simulink model "Assignment_2_PacemakerProj"  (R2022b)
settings: Solver=FixedStepAuto  StartTime=0.0  StopTime=100  FixedStep=1e-3  RelTol=1e-3  EnableMultiTasking=on
undefined symbols (not defined in the file): D0, D1, D10, D11, D12, D13, D2, D3, D4, D5, D6, D7, D8, D9, PTA0, PTA1, PTA2, PTB23, PTB9, PTC16, PTC17, PTC2, PTC3, PTC4, PTD0, PTD1, PTD2, PTD3
libraries: frdmk64flib x24, etargetslib x3, simulink x3
settings Model: ExtModeTrigDuration=5  Creator=varun  LastModifiedBy=lupas
settings OptimizationCC: EnhancedBackFolding=on  PassReuseOutputArgsAs=Individual arguments  ZeroExternalMemoryAtStartup=off  ZeroInternalMemoryAtStartup=off  MaxStackSize=64  OptimizeBlockOrder=speed  DifferentSizesBufferReuse=on  OptimizationCustomize=off  EfficientTunableParamExpr=on
settings DebuggingCC: ParameterTunabilityLossMsg=error
settings HardwareCC: ProdBitPerPointer=32  ProdBitPerSizeT=32  ProdBitPerPtrDiffT=32  ProdLargestAtomicInteger=Long  ProdLargestAtomicFloat=Double  ProdWordSize=32  ProdHWDeviceType=ARM Compatible->ARM Cortex
settings SFSimCC: MATLABDynamicMemAlloc=off
settings RTWCC: Description=Embedded Coder  SystemTargetFile=ert.tlc  HardwareBoard=NXP FRDM-K64F  TLCOptions="-aInlineSetEventsForThisBaseRateFcn=TLC_FALSE -aSuppressMultiTaskScheduler=TLC_FALSE  -aRateBasedStepFcn=0"  TemplateMakefile=ert_default_tmf  Toolchain=GNU Tools for ARM Embedded Processors
settings CodeAppCC: ForceParamTrailComments=on  IgnoreCustomStorageClasses=off  OperatorAnnotations=on  SimulinkDataObjDesc=on  SFDataObjDesc=on  InsertBlockDesc=on
settings ERTTargetCC: ExtModeTransport=4  ExtModeMexFile=sendToCommService

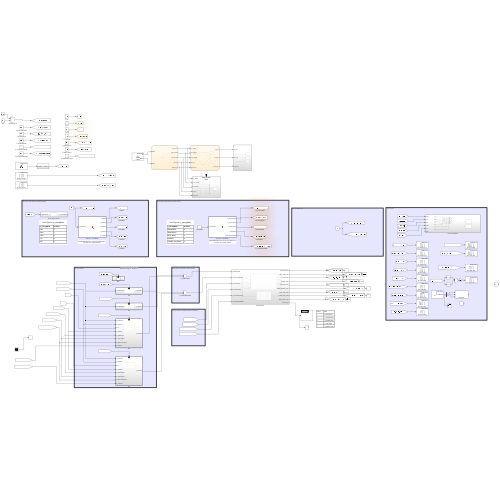
[thumbnail: Simulink's stored preview of the top-level diagram]
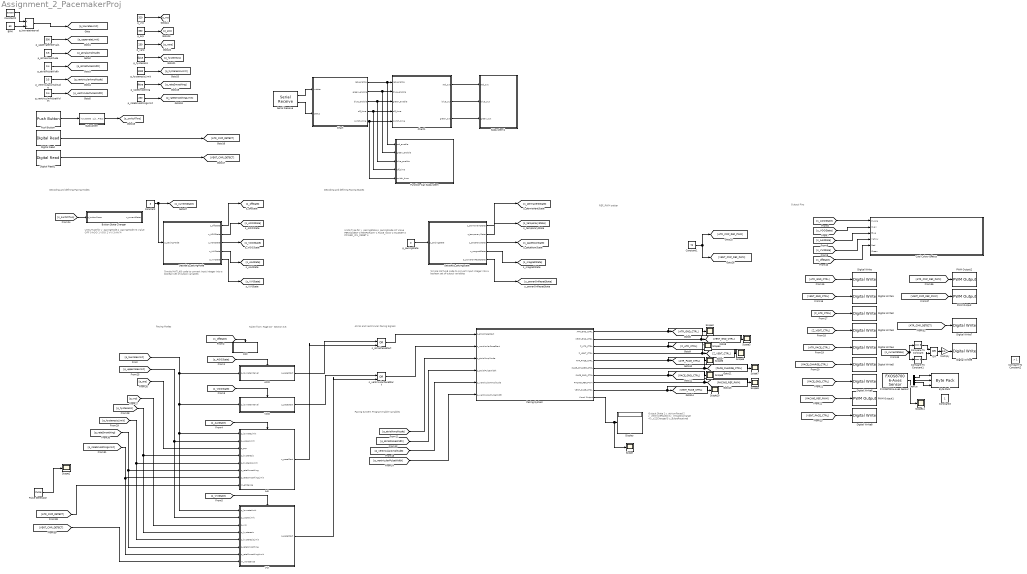
== system Assignment_2_PacemakerProj ==
  note: REF_PWM setter
  note: Output Pins
  note: Pacing System Programmable Variables
  note: Output
      | State
      |
      | 1
      | y_atriumPaced
      |
      | 2
      | y_ventriclePaced
      |
      | 3
      | y_initialDischarge
      |
      | 4
      | y_c22Charged
      |
      | 5
      | y_pulseReceived
  note: Atrial and Ventricular Pacing Signals
  note: Decoding and defining Pacing States
  note: Decoding and defining Pacing Modes
  note: Simple MATLAB code to convert input integer into a boolean set of output variables
  note: Taken from: Page 16 - Section 3.5
  note: Units/Type for y_pacingMode
      |
      | p_pacingMode
      | Int Value
      |
      | OFF
      | 0
      |
      | AOO
      | 1
      |
      | VOO
      | 2
      |
      | VVI
      | 3
      |
      | AAI
      | 4
  note: Pacing Modes
  note: Units/Type for y_pacingState
      |
      | p_pacingMode
      | Int Value
      |
      | PERMANENT
      | 0
      |
      | TEMPORARY
      | 1
      |
      | PACE_NOW
      | 2
      |
      | MAGNET
      | 3
      |
      | POWER_ON_RESET
      | 4
  note: Simple MATLAB code to convert input integer into a boolean set of output variables
  AAI : Subsystem
  AOO : Subsystem
  BPM : Constant  Value=60
  Button State Changer : Subsystem
  Byte Pack : etargetslib/Byte Pack  datatypes={'double', 'double', 'double'}  byteAlign=1
  Chart : Stateflow chart  TreatAsAtomicUnit=on
  Chart1 : Stateflow chart  TreatAsAtomicUnit=on
  Compare To Constant : simulink/Logic and Bit Operations/Compare To Constant  relop===  const=3  OutDataTypeStr=boolean
  Compare To Constant1 : simulink/Logic and Bit Operations/Compare To Constant  relop===  const=4  OutDataTypeStr=boolean
  Compare To Constant2 : simulink/Logic and Bit Operations/Compare To Constant  relop=>  const=1  OutDataTypeStr=boolean
  Constant : Constant  Value=3
  Constant1 : Constant  Value=70
  Constant2 : Constant  Value=60000
  Constant3 : Constant
  Cool Colour Effects : Subsystem
  Decode p_pacingMode : MATLAB Function  TreatAsAtomicUnit=on
  Decode p_pacingState : MATLAB Function  TreatAsAtomicUnit=on
  Demux : Demux  Outputs=3
  Digital Read : frdmk64flib/Digital Read  Whichpin=PTC16 (D0)  SampleTime=-1
  Digital Read1 : frdmk64flib/Digital Read  Whichpin=PTC17 (D1)  SampleTime=-1
  Digital Write : frdmk64flib/Digital Write  Whichpin=PTD2 (D11)
  Digital Write1 : frdmk64flib/Digital Write  Whichpin=PTD3 (D12)
  Digital Write2 : frdmk64flib/Digital Write  Whichpin=PTB23 (D4)
  Digital Write3 : frdmk64flib/Digital Write  Whichpin=PTC3 (D7)
  Digital Write4 : frdmk64flib/Digital Write  Whichpin=PTA0 (D8)
  Digital Write5 : frdmk64flib/Digital Write  Whichpin=PTB9 (D2)
  Digital Write6 : frdmk64flib/Digital Write  Whichpin=PTD0 (D10)
  Digital Write7 : frdmk64flib/Digital Write  Whichpin=RED_LED
  Digital Write8 : frdmk64flib/Digital Write  Whichpin=PTC4 (D9)
  Digital Write9 : frdmk64flib/Digital Write  Whichpin=PTD1 (D13)
  Display : Display
  FXOS8700 6-Axes Sensor : frdmk64flib/FXOS8700 6-Axes Sensor  Activesensor=Accelerometer only  ODR=400Hz  HybridODR=400Hz  Accelfullrange=-4g to +4g  SampleTime=-1
  Function-Call Subsystem : Subsystem  TreatAsAtomicUnit=on
  Multiply : Gain  Gain=3.3  OutDataTypeStr=double
  OFF : Subsystem
  OR : Logic  Operator=OR  IconShape=distinctive  AllPortsSameDT=off  OutDataTypeStr=boolean
  PWM Output : frdmk64flib/PWM Output  Whichpin=PTA1 (D3)  InitialFrequency=2000  InitialDutyCycle=50
  PWM Output1 : frdmk64flib/PWM Output  Whichpin=PTA2 (D5)  InitialFrequency=2000  InitialDutyCycle=50
  PWM Output2 : frdmk64flib/PWM Output  Whichpin=PTC2 (D6)  InitialFrequency=2000  InitialDutyCycle=50
  Pacing System : Subsystem
  Pulse Generator : DiscretePulseGenerator  PulseType=Time based  Amplitude=3.5  PulseWidth=0.5
  Push Button : frdmk64flib/Push Button  Whichswitch=SW2  SampleTime1=-1
  Scope{,1..11} (12 alike) : Scope
  Serial Receive : frdmk64flib/Serial Receive  SCIModule=0  Baudrate=uint32(9600)  Parity=None  StopBits=1  HardwareFlowControl=None  ByteOrder=LittleEndian  DataType=uint8  DataLength=11  BlockingMode=off  OutputStatus=on  SampleTime=0.1
  Subsystem : Subsystem
  Subsystem1 : Subsystem
  VOO : Subsystem
  VVI : Subsystem
  p_arp : Constant  Value=350  OutDataTypeStr=int16
  p_atrialAmplitude : Constant  Value=3.5  OutDataTypeStr=double
  p_atrialPulseWidth : Constant  Value=0.4  OutDataTypeStr=double
  p_hysteresis : Constant  Value=false  OutDataTypeStr=boolean
  p_hysteresisLimit : Constant  Value=1000  OutDataTypeStr=int16
  p_lowrateInterval : Product  Inputs=*/
  p_pacingState : Constant  Value=0
  p_rateSmoothing : Constant  Value=false  OutDataTypeStr=boolean
  p_rateSmoothingLimit : Constant  Value=250  OutDataTypeStr=uint16
  p_upperrateInterval1 : Constant  Value=500  OutDataTypeStr=int16
  p_varp : Constant  Value=250  OutDataTypeStr=int16
  p_ventricularAmplitude : Constant  Value=3.5  OutDataTypeStr=double
  p_ventricularPulseWidth : Constant  Value=0.4  OutDataTypeStr=double
  p_vrp : Constant  Value=320  OutDataTypeStr=int16
  s_atrialPaceStart : Logic  Operator=OR  IconShape=distinctive  AllPortsSameDT=off  OutDataTypeStr=boolean
  s_ventricularPaceStart : Logic  Operator=OR  IconShape=distinctive  AllPortsSameDT=off  OutDataTypeStr=boolean
  wires:
  [s_offState] -> OFF/Enable
  Decode p_pacingMode/1(s_offState) -> [s_offState]
  Decode p_pacingMode/2(s_AOOState) -> [s_AOOState]
  Decode p_pacingMode/4(s_AAIState) -> [s_AAIState]
  Decode p_pacingMode/5(S_VVIState) -> [s_VVIState]
  Decode p_pacingMode/3(s_VOOState) -> [s_VOOState]
  p_pacingState/1 -> Decode p_pacingState/1(p_pacingState)
  Decode p_pacingState/1(s_permanentState) -> [s_permanentState]
  Decode p_pacingState/2(s_temporaryState) -> [s_temporaryState]
  Decode p_pacingState/3(s_paceNowState) -> [s_paceNowState]
  Decode p_pacingState/4(s_magnetState) -> [s_magnetState]
  Decode p_pacingState/5(S_powerOnResetState) -> [s_powerOnResetState]
  AAI/1(s_paceStart) -> s_atrialPaceStart/2
  VVI/1(s_paceStart) -> s_ventricularPaceStart/2
  [s_AAIState] -> AAI/Enable
  [s_VVIState] -> VVI/Enable
  [s_AOOState] -> Cool Colour Effects/1(Purple)
  [s_VOOState] -> Cool Colour Effects/2(Cyan)
  [s_AAIState] -> Cool Colour Effects/3(Blue)
  [s_VVIState] -> Cool Colour Effects/4(Yellow)
  [s_offState] -> Cool Colour Effects/5(Red)
  p_upperrateInterval1/1 -> [p_upperrateLimit]
  p_atrialAmplitude/1 -> [p_atrialAmplitude]
  p_atrialPulseWidth/1 -> [p_atrialPulseWidth]
  p_ventricularAmplitude/1 -> [p_ventricularAmplitude]
  p_ventricularPulseWidth/1 -> [p_ventricularPulseWidth]
  s_atrialPaceStart/1 -> Pacing System/1(s_atrialPaceStart)
  [p_atrialAmplitude] -> Pacing System/3(p_atrialAmplitude)
  [p_atrialPulseWidth] -> Pacing System/4(p_atrialPulseWidth)
  [p_ventricularAmplitude] -> Pacing System/5(p_ventricularAmplitude)
  [p_ventricularPulseWidth] -> Pacing System/6(p_ventricularPulseWidth)
  s_ventricularPaceStart/1 -> Pacing System/2(s_ventricularPaceStart)
  Pacing System/1(ATR_GND_CTRL) -> [ATR_GND_CTRL], Scope2/1
  Pacing System/3(Z_ATR_CTRL) -> [Z_ATR_CTRL], Scope4/1
  Pacing System/2(VENT_GND_CTRL) -> [VENT_GND_CTRL], Scope3/1
  Pacing System/4(Z_VENT_CTRL) -> Scope5/1, [Z_VENT_CTRL]
  Pacing System/6(PACE_CHARGE_CTRL) -> Scope7/1, [PACE_CHARGE_CTRL]
  Pacing System/5(ATR_PACE_CTRL) -> [ATR_PACE_CTRL], Scope6/1
  Pacing System/7(PACE_GND_CTRL) -> Scope8/1, [PACE_GND_CTRL]
  Pacing System/9(VENT_PACE_CTRL) -> [VENT_PACE_CTRL], Scope10/1
  Pacing System/8(PACING_REF_PWM) -> Scope9/1, [PACING_REF_PWM]
  Pacing System/10(Visual Output) -> Scope/1, Display/1
  [VENT_PACE_CTRL] -> Digital Write8/1
  [PACING_REF_PWM] -> PWM Output1/1
  [PACE_GND_CTRL] -> Digital Write6/1
  [PACE_CHARGE_CTRL] -> Digital Write5/1
  [ATR_PACE_CTRL] -> Digital Write4/1
  [Z_VENT_CTRL] -> Digital Write3/1
  [Z_ATR_CTRL] -> Digital Write2/1
  [VENT_GND_CTRL] -> Digital Write1/1
  [ATR_GND_CTRL] -> Digital Write/1
  Push Button/1 -> Subsystem/1(inputState)
  Subsystem/1(s_buttonPress) -> [s_switchTwo]
  [s_switchTwo] -> Button State Changer/1(s_buttonPress)
  [s_AOOState] -> AOO/Enable
  [s_VOOState] -> VOO/Enable
  [p_lowrateLimit] -> VVI/1(p_lowrateLimit), AAI/1(p_lowrateLimit), VOO/1(p_lowrateInterval), AOO/1(p_lowrateInterval)
  AOO/1(s_paceStart) -> s_atrialPaceStart/1
  VOO/1(s_paceStart) -> s_ventricularPaceStart/1
  p_rateSmoothingLimit/1 -> [p_rateSmoothingLimit]
  p_rateSmoothing/1 -> [p_rateSmoothing]
  p_hysteresisLimit/1 -> [p_hysteresisLimit]
  p_hysteresis/1 -> [p_hysteresis]
  p_vrp/1 -> [p_vrp]
  p_arp/1 -> [p_arp]
  p_varp/1 -> [p_varp]
  [p_upperrateLimit] -> VVI/2(p_upperLimit), AAI/2(p_upperLimit)
  [p_arp] -> AAI/3(p_arp)
  [p_vrp] -> VVI/3(p_vrp)
  [p_hysteresis] -> VVI/4(p_hysteresis), AAI/4(p_hysteresis)
  [p_hysteresisLimit] -> VVI/5(p_hysteresisLimit), AAI/5(p_hystersisLimit)
  [p_rateSmoothing] -> VVI/6(p_rateSmoothing), AAI/6(p_rateSmoothing)
  [p_rateSmoothingLimit] -> VVI/7(p_rateSmoothingLimit), AAI/7(p_rateSmoothingLimit)
  Digital Read/1 -> [ATR_CMP_DETECT]
  Digital Read1/1 -> [VENT_CMP_DETECT]
  [ATR_CMP_REF_PWM] -> PWM Output2/1
  [VENT_CMP_REF_PWM] -> PWM Output/1
  [VENT_CMP_DETECT] -> VVI/8(m_ventSense)
  BPM/1 -> p_lowrateInterval/2
  p_lowrateInterval/1 -> [p_lowrateLimit]
  Constant2/1 -> p_lowrateInterval/1
  Constant1/1 -> [ATR_CMP_REF_PWM], [VENT_CMP_REF_PWM]
  Constant/1 -> Decode p_pacingMode/1(p_pacingMode), [s_currentState]
  OR/1 -> Multiply/1
  Compare To Constant/1 -> OR/1
  Compare To Constant1/1 -> OR/2
  Multiply/1 -> Digital Write9/1
  Pulse Generator/1 -> Scope1/1
  [s_currentState] -> Compare To Constant1/1, Compare To Constant/1
  [ATR_CMP_DETECT] -> AAI/8(m_atrSense)
  Demux/1 -> Byte Pack/1
  Demux/2 -> Byte Pack/2
  Demux/3 -> Byte Pack/3
  FXOS8700 6-Axes Sensor/1 -> Scope11/1
  [ATR_CMP_DETECT] -> Digital Write7/1
  Serial Receive/1 -> Chart/1(rxdata)
  Serial Receive/2 -> Chart/2(status)
  Chart/1(red_enable) -> Function-Call Subsystem/1(red_enable), Chart1/1(red_enable)
  Chart/2(green_enable) -> Function-Call Subsystem/2(green_enable), Chart1/2(blue_enable)
  Chart/3(blue_enable) -> Function-Call Subsystem/3(blue_enable), Chart1/3(green_enable)
  Chart/4(off_time) -> Function-Call Subsystem/4(off_time), Chart1/4(off_time)
  Chart/5(switch_time) -> Function-Call Subsystem/5(switch_time), Chart1/5(switch_time)
  Chart1/1(red_out) -> Subsystem1/1(red_out)
  Chart1/2(blue_out) -> Subsystem1/2(blue_out)
  Chart1/3(green_out) -> Subsystem1/3(green_out)

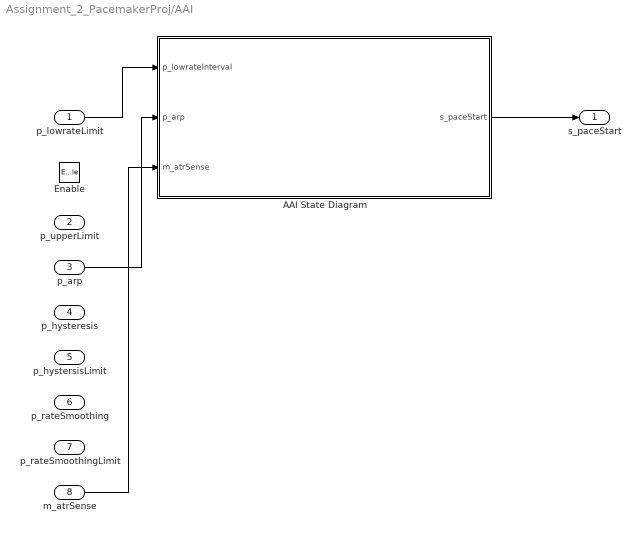
== system Assignment_2_PacemakerProj/AAI ==
  p_lowrateLimit : Inport
  p_upperLimit : Inport  Port=2
  p_arp : Inport  Port=3
  p_hysteresis : Inport  Port=4
  p_hystersisLimit : Inport  Port=5
  p_rateSmoothing : Inport  Port=6
  p_rateSmoothingLimit : Inport  Port=7
  m_atrSense : Inport  Port=8
  Enable : EnablePort
  AAI State Diagram : Stateflow chart  TreatAsAtomicUnit=on
  s_paceStart : Outport
  wires:
  p_lowrateLimit/1 -> AAI State Diagram/1(p_lowrateInterval)
  AAI State Diagram/1(s_paceStart) -> s_paceStart/1
  m_atrSense/1 -> AAI State Diagram/3(m_atrSense)
  p_arp/1 -> AAI State Diagram/2(p_arp)

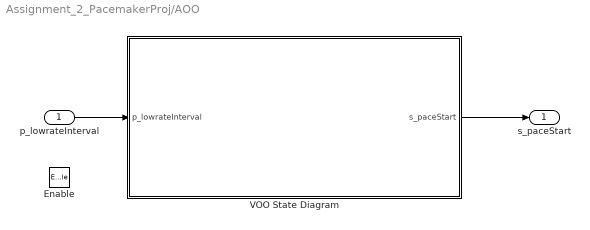
== system Assignment_2_PacemakerProj/AOO ==
  p_lowrateInterval : Inport
  Enable : EnablePort
  VOO State Diagram : Stateflow chart  TreatAsAtomicUnit=on
  s_paceStart : Outport
  wires:
  p_lowrateInterval/1 -> VOO State Diagram/1(p_lowrateInterval)
  VOO State Diagram/1(s_paceStart) -> s_paceStart/1

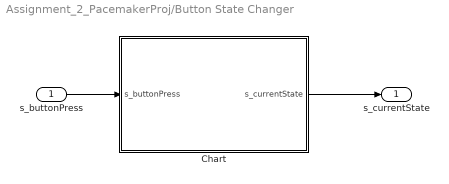
== system Assignment_2_PacemakerProj/Button State Changer ==
  s_buttonPress : Inport  OutDataTypeStr=boolean
  Chart : Stateflow chart  TreatAsAtomicUnit=on
  s_currentState : Outport
  wires:
  s_buttonPress/1 -> Chart/1(s_buttonPress)
  Chart/1(s_currentState) -> s_currentState/1

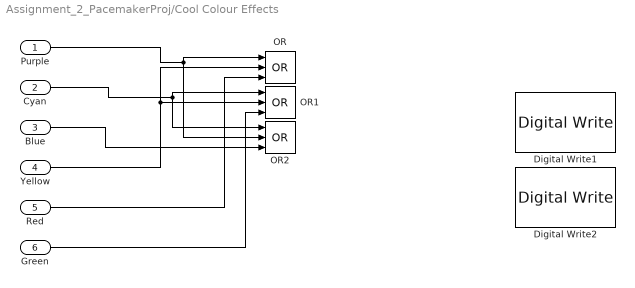
== system Assignment_2_PacemakerProj/Cool Colour Effects ==
  Purple : Inport
  Cyan : Inport  Port=2
  Blue : Inport  Port=3
  Yellow : Inport  Port=4
  Red : Inport  Port=5
  Green : Inport  Port=6
  Digital Write1 : frdmk64flib/Digital Write  Whichpin=GREEN_LED
  Digital Write2 : frdmk64flib/Digital Write  Whichpin=BLUE_LED
  OR : Logic  Operator=OR  Inputs=3  IconShape=distinctive  AllPortsSameDT=off  OutDataTypeStr=boolean
  OR1 : Logic  Operator=OR  Inputs=3  IconShape=distinctive  AllPortsSameDT=off  OutDataTypeStr=boolean
  OR2 : Logic  Operator=OR  Inputs=3  IconShape=distinctive  AllPortsSameDT=off  OutDataTypeStr=boolean
  wires:
  Blue/1 -> OR2/3
  Cyan/1 -> OR2/1, OR1/1
  Purple/1 -> OR2/2, OR/1
  Yellow/1 -> OR1/2, OR/2
  Red/1 -> OR/3
  Green/1 -> OR1/3

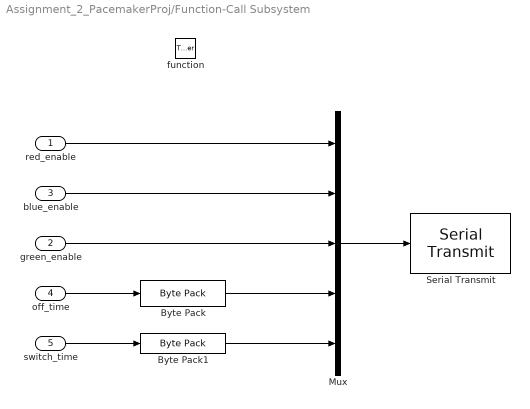
== system Assignment_2_PacemakerProj/Function-Call Subsystem ==
  red_enable : Inport
  green_enable : Inport  Port=2
  blue_enable : Inport  Port=3
  off_time : Inport  Port=4
  switch_time : Inport  Port=5
  function : TriggerPort  TriggerType=function-call  IsSimulinkFunction=on  FunctionName=send_params  VariantControl=(inherit)
  Byte Pack : etargetslib/Byte Pack  datatypes={'single'}  byteAlign=1
  Byte Pack1 : etargetslib/Byte Pack  datatypes={'uint16'}  byteAlign=1
  Mux : Mux  Inputs=5
  Serial Transmit : frdmk64flib/Serial Transmit  SCIModule=0  Baudrate=uint32(9600)  Parity=None  StopBits=1  HardwareFlowControl=None  ByteOrder=LittleEndian  BlockingMode=on  OutputStatus=off
  wires:
  switch_time/1 -> Byte Pack1/1
  green_enable/1 -> Mux/3
  blue_enable/1 -> Mux/2
  Mux/1 -> Serial Transmit/1
  off_time/1 -> Byte Pack/1
  Byte Pack1/1 -> Mux/5
  Byte Pack/1 -> Mux/4
  red_enable/1 -> Mux/1

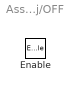
== system Assignment_2_PacemakerProj/OFF ==
  Enable : EnablePort

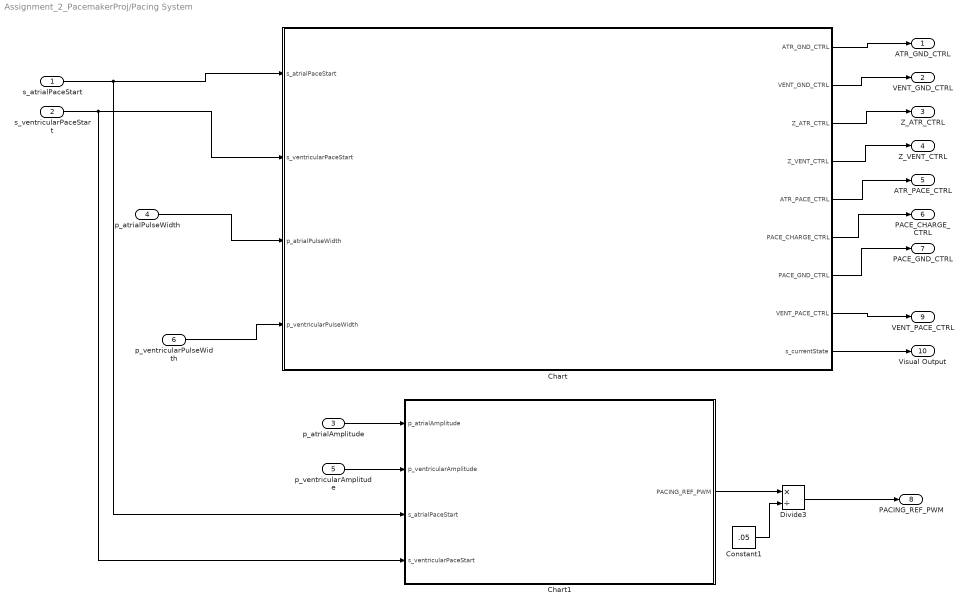
== system Assignment_2_PacemakerProj/Pacing System ==
  s_atrialPaceStart : Inport
  s_ventricularPaceStart : Inport  Port=2
  p_atrialAmplitude : Inport  Port=3
  p_atrialPulseWidth : Inport  Port=4
  p_ventricularAmplitude : Inport  Port=5  OutDataTypeStr=double
  p_ventricularPulseWidth : Inport  Port=6  OutDataTypeStr=double
  Chart : Stateflow chart  TreatAsAtomicUnit=on
  Chart1 : Stateflow chart  TreatAsAtomicUnit=on
  Constant1 : Constant  Value=.05  OutDataTypeStr=double
  Divide3 : Product  Inputs=*/
  ATR_GND_CTRL : Outport
  VENT_GND_CTRL : Outport  Port=2
  Z_ATR_CTRL : Outport  Port=3
  Z_VENT_CTRL : Outport  Port=4
  ATR_PACE_CTRL : Outport  Port=5
  PACE_CHARGE_CTRL : Outport  Port=6
  PACE_GND_CTRL : Outport  Port=7
  PACING_REF_PWM : Outport  Port=8
  VENT_PACE_CTRL : Outport  Port=9
  Visual Output : Outport  Port=10
  wires:
  s_atrialPaceStart/1 -> Chart1/3(s_atrialPaceStart), Chart/1(s_atrialPaceStart)
  s_ventricularPaceStart/1 -> Chart1/4(s_ventricularPaceStart), Chart/2(s_ventricularPaceStart)
  p_atrialPulseWidth/1 -> Chart/3(p_atrialPulseWidth)
  Chart/1(ATR_GND_CTRL) -> ATR_GND_CTRL/1
  Chart/2(VENT_GND_CTRL) -> VENT_GND_CTRL/1
  Chart/3(Z_ATR_CTRL) -> Z_ATR_CTRL/1
  Chart/4(Z_VENT_CTRL) -> Z_VENT_CTRL/1
  Chart/5(ATR_PACE_CTRL) -> ATR_PACE_CTRL/1
  Chart/6(PACE_CHARGE_CTRL) -> PACE_CHARGE_CTRL/1
  Chart/7(PACE_GND_CTRL) -> PACE_GND_CTRL/1
  Chart/8(VENT_PACE_CTRL) -> VENT_PACE_CTRL/1
  Chart/9(s_currentState) -> Visual Output/1
  p_ventricularPulseWidth/1 -> Chart/4(p_ventricularPulseWidth)
  p_ventricularAmplitude/1 -> Chart1/2(p_ventricularAmplitude)
  p_atrialAmplitude/1 -> Chart1/1(p_atrialAmplitude)
  Chart1/1(PACING_REF_PWM) -> Divide3/1
  Constant1/1 -> Divide3/2
  Divide3/1 -> PACING_REF_PWM/1

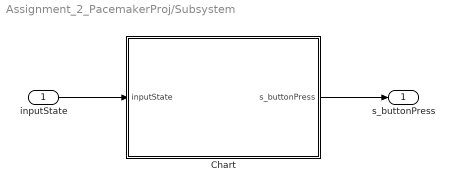
== system Assignment_2_PacemakerProj/Subsystem ==
  inputState : Inport
  Chart : Stateflow chart  TreatAsAtomicUnit=on
  s_buttonPress : Outport
  wires:
  inputState/1 -> Chart/1(inputState)
  Chart/1(s_buttonPress) -> s_buttonPress/1

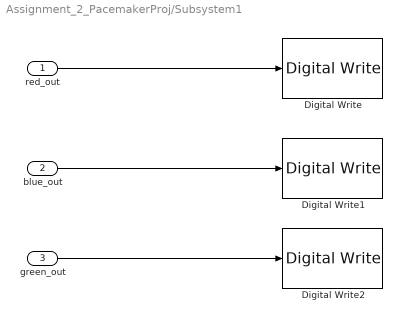
== system Assignment_2_PacemakerProj/Subsystem1 ==
  red_out : Inport
  blue_out : Inport  Port=2
  green_out : Inport  Port=3
  Digital Write : frdmk64flib/Digital Write  Whichpin=RED_LED
  Digital Write1 : frdmk64flib/Digital Write  Whichpin=GREEN_LED
  Digital Write2 : frdmk64flib/Digital Write  Whichpin=BLUE_LED
  wires:
  red_out/1 -> Digital Write/1
  blue_out/1 -> Digital Write1/1
  green_out/1 -> Digital Write2/1

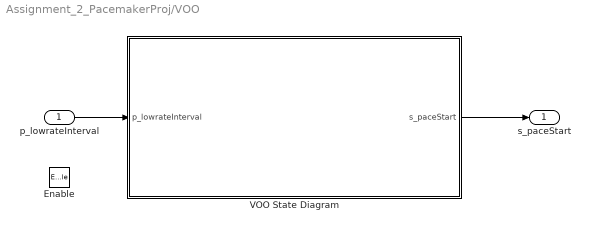
== system Assignment_2_PacemakerProj/VOO ==
  p_lowrateInterval : Inport
  Enable : EnablePort
  VOO State Diagram : Stateflow chart  TreatAsAtomicUnit=on
  s_paceStart : Outport
  wires:
  p_lowrateInterval/1 -> VOO State Diagram/1(p_lowrateInterval)
  VOO State Diagram/1(s_paceStart) -> s_paceStart/1

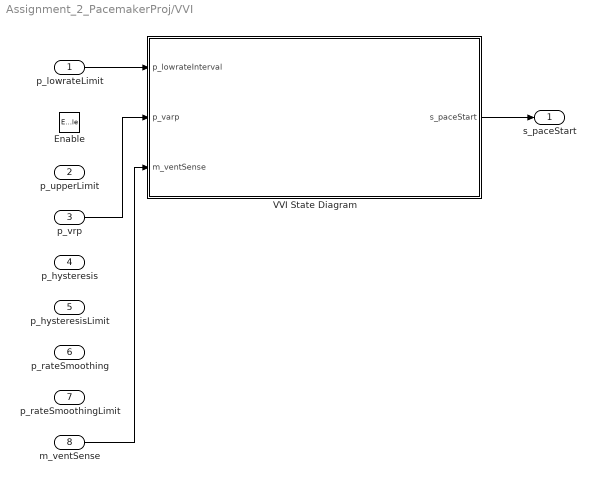
== system Assignment_2_PacemakerProj/VVI ==
  p_lowrateLimit : Inport
  p_upperLimit : Inport  Port=2
  p_vrp : Inport  Port=3
  p_hysteresis : Inport  Port=4
  p_hysteresisLimit : Inport  Port=5
  p_rateSmoothing : Inport  Port=6
  p_rateSmoothingLimit : Inport  Port=7
  m_ventSense : Inport  Port=8
  Enable : EnablePort
  VVI State Diagram : Stateflow chart  TreatAsAtomicUnit=on
  s_paceStart : Outport
  wires:
  p_lowrateLimit/1 -> VVI State Diagram/1(p_lowrateInterval)
  VVI State Diagram/1(s_paceStart) -> s_paceStart/1
  p_vrp/1 -> VVI State Diagram/2(p_varp)
  m_ventSense/1 -> VVI State Diagram/3(m_ventSense)

== matlab function Assignment_2_PacemakerProj/Decode p_pacingState ==
  data: p_pacingState input; s_permanentState output; s_temporaryState output; s_paceNowState output; s_magnetState output; S_powerOnResetState output
function [s_permanentState,s_temporaryState, s_paceNowState, s_magnetState, S_powerOnResetState] = decodeInputInteger(p_pacingState)

stateList = zeros(1,5);

stateList(p_pacingState + 1) = 1;

s_permanentState = stateList(1);
s_temporaryState = stateList(2);
s_paceNowState = stateList(3);
s_magnetState = stateList(4);
S_powerOnResetState = stateList(5);

== stateflow chart Assignment_2_PacemakerProj/Pacing System/Chart ==
  note: Step 1
  state chargingPrimaryCapacitor
    entry:
    % As per Section 3.3.1
    % To ensure atr/vent are discharged
    % upon initial start
    ATR_PACE_CTRL = false;
    VENT_PACE_CTRL = false;
    PACE_CHARGE_CTRL = true;
    PACE_GND_CTRL=true;
  state initalState
    entry:
    % x_GND_CTRL is disabled
    ATR_GND_CTRL = false;
    VENT_GND_CTRL = false;
    % Z_x_CTRL is also disabled
    Z_ATR_CTRL = false;
    Z_VENT_CTRL = false;
  state chargingBuffer
    exit:
    s_currentState = 4; % y_c22Charged
  state pacingBuffer
    exit:
    s_currentState = 5; % y_pulseReceived
  note: Step 2
  state atrialPacing
    entry:
    % As per Section 3.3.2
    PACE_CHARGE_CTRL = false;
    % PACE_GND_CTRL = true;
    ATR_PACE_CTRL = true;
    ATR_GND_CTRL = false;
    Z_ATR_CTRL = false;
    Z_VENT_CTRL = false;
    VENT_GND_CTRL = false;
    VENT_PACE_CTRL = false;
    exit:
    s_currentState = 1; % y_atriumPaced
  state ventricularPacing
    entry:
    % As per Section 3.3.2
    PACE_CHARGE_CTRL = false;
    % PACE_GND_CTRL = true;
    ATR_PACE_CTRL = false;
    ATR_GND_CTRL = false;
    Z_ATR_CTRL = false;
    Z_VENT_CTRL = false;
    VENT_GND_CTRL = false;
    VENT_PACE_CTRL = true;
    exit:
    s_currentState = 2; % y_ventriclePaced
  state dischargingAtrialBlockCapacitor
    entry:
    % Do steps common to Step 3 and Step 1 here
    % PACE_GND_CTRL = true;
    % VENT_PACE_CTRL = false;
    % Z_ATR_CTRL = false;
    % Z_VENT_CTRL = false;
    ATR_PACE_CTRL = false;
    % Step unique to ventricular pacing
    % VENT_GND_CTRL = false;
    ATR_GND_CTRL = true;
    exit:
    s_currentState = 3; % y_initialDischarge
  note: Step 3
  state dischargingVentricularBlockCapacitor
    entry:
    % Do steps common to Step 3 and Step 1 here
    % PACE_GND_CTRL = true;
    VENT_PACE_CTRL = false;
    % Z_ATR_CTRL = false;
    % Z_VENT_CTRL = false;
    % ATR_PACE_CTRL = false;
    % ATR_GND_CTRL = false;
    % Step unique to ventricular pacing
    % ATR_GND_CTRL = false;
    VENT_GND_CTRL = true;
    exit:
    s_currentState = 3; % y_initialDischarge
  pacingBuffer -> ventricularPacing [order 2] : [s_atrialPaceStart == false && s_ventricularPaceStart == true]
  (default) -> initalState
  initalState -> chargingPrimaryCapacitor
  pacingBuffer -> atrialPacing [order 1] : [s_atrialPaceStart == true && s_ventricularPaceStart == false]
  chargingPrimaryCapacitor -> chargingBuffer : [s_atrialPaceStart == false && s_ventricularPaceStart == false]
  chargingBuffer -> pacingBuffer
  dischargingVentricularBlockCapacitor -> chargingPrimaryCapacitor
  dischargingAtrialBlockCapacitor -> chargingPrimaryCapacitor
  atrialPacing -> dischargingAtrialBlockCapacitor : after(p_atrialPulseWidth,msec)
  ventricularPacing -> dischargingVentricularBlockCapacitor : after(p_ventricularPulseWidth,msec)
  data: ATR_GND_CTRL output; VENT_GND_CTRL output; Z_ATR_CTRL output; Z_VENT_CTRL output; ATR_PACE_CTRL output; PACE_CHARGE_CTRL output; PACE_GND_CTRL output; VENT_PACE_CTRL output; s_atrialPaceStart input; s_ventricularPaceStart input; p_atrialPulseWidth input; p_ventricularPulseWidth input; s_currentState output

== stateflow chart Assignment_2_PacemakerProj/Pacing System/Chart1 ==
  state initialState
    entry:
    PACING_REF_PWM = 0;
  state atrialPacing
    entry:
    PACING_REF_PWM = p_atrialAmplitude;
  state ventricularPacing
    entry:
    PACING_REF_PWM = p_ventricularAmplitude;
  (default) -> initialState
  initialState -> atrialPacing [order 1] : [s_atrialPaceStart == true && s_ventricularPaceStart == false]
  initialState -> ventricularPacing [order 2] : [s_atrialPaceStart == false && s_ventricularPaceStart == true]
  atrialPacing -> ventricularPacing : [s_atrialPaceStart == false && s_ventricularPaceStart == true]
  ventricularPacing -> atrialPacing : [s_atrialPaceStart == true && s_ventricularPaceStart == false]
  data: PACING_REF_PWM output; p_atrialAmplitude input; p_ventricularAmplitude input; s_atrialPaceStart input; s_ventricularPaceStart input

== stateflow chart Assignment_2_PacemakerProj/Subsystem/Chart ==
  state stillState
    entry:
    s_buttonPress = false;
  state buttonPressed
    entry:
    s_buttonPress = true;
  (default) -> stillState
  stillState -> buttonPressed : [inputState == true]
  buttonPressed -> stillState : after(1,sec)
  data: inputState input; s_buttonPress output

== stateflow chart Assignment_2_PacemakerProj/VOO/VOO State Diagram ==
  state NO_PACE
    entry:
    s_paceStart = true;
  state PACE
    entry:
    s_paceStart = false;
  (default) -> NO_PACE
  PACE -> NO_PACE : after(p_lowrateInterval, msec)
  NO_PACE -> PACE : after(1, msec)
  data: p_lowrateInterval input; s_paceStart output

== stateflow chart Assignment_2_PacemakerProj/AAI/AAI State Diagram ==
  state PACE
    entry:
    s_paceStart = true;
  state NO_PACE
    entry:
    s_paceStart = false;
  state ATR_REF
    entry:
    s_paceStart = false;
  (default) -> NO_PACE
  NO_PACE -> PACE [order 2] : [after(p_lowrateInterval, msec)]
  ATR_REF -> NO_PACE : after(p_arp, msec)
  PACE -> ATR_REF : after(1, msec)
  NO_PACE -> ATR_REF [order 1] : [m_atrSense >= 1]
  data: p_lowrateInterval input; p_arp input; s_paceStart output; m_atrSense input

== stateflow chart Assignment_2_PacemakerProj/VVI/VVI State Diagram ==
  state PACE
    entry:
    s_paceStart = true;
  state NO_PACE
    entry:
    s_paceStart = false;
  state VENT_REF
    entry:
    s_paceStart = false;
  (default) -> NO_PACE
  NO_PACE -> PACE [order 1] : [after(p_lowrateInterval, msec)]
  VENT_REF -> NO_PACE : after(p_varp, msec)
  PACE -> VENT_REF : after(1, msec)
  NO_PACE -> VENT_REF [order 2] : [m_ventSense >= 1]
  data: p_lowrateInterval input; p_varp input; s_paceStart output; m_ventSense input

== stateflow chart Assignment_2_PacemakerProj/Chart ==
  state SET_PARAM
    entry:
    red_enable = rxdata(3);
    green_enable = rxdata(4);
    blue_enable = rxdata(5);
    off_time = typecast(rxdata(6:9), 'single');
    switch_time = typecast(rxdata(10:11), 'uint16');
  state INITIAL
    entry:
    red_enable = 1;
    green_enable = 1;
    blue_enable = 0;
    off_time = 0.5;
    switch_time = 200;
  state STANDBY
  state ECHO_PARAM
    entry:
    send_params();
  SET_PARAM -> STANDBY
  (default) -> INITIAL
  (junction 14) -> SET_PARAM [order 1] : [rxdata(2) == hex2dec('55')]
  (junction 12) -> STANDBY [order 2]
  INITIAL -> STANDBY
  STANDBY -> (junction 12) : [status==0]
  (junction 12) -> (junction 14) [order 1] : [rxdata(1) == hex2dec('16')]
  (junction 14) -> ECHO_PARAM [order 2] : [rxdata(2) == hex2dec('22')]
  ECHO_PARAM -> STANDBY
  data: rxdata input; status input; red_enable output; green_enable output; blue_enable output; off_time output; switch_time output

== stateflow chart Assignment_2_PacemakerProj/Chart1 ==
  settings: executeAtInitialization=1
  state OFF
    entry:
    red_out = 0;
    blue_out = 0;
    green_out = 0;
  state RED_ON
    entry:
    red_out = 1;
    green_out = 0;
    blue_out = 0;
  state BLUE_ON
    entry:
    red_out = 0;
    green_out = 0;
    blue_out = 1;
  state GREEN_ON
    entry:
    red_out = 0;
    green_out = 1;
    blue_out = 0;
  (default) -> OFF
  OFF -> (junction 6) : after(off_time, sec)
  (junction 6) -> RED_ON [order 1] : [red_enable == 1]
  (junction 6) -> (junction 7) [order 2]
  (junction 9) -> OFF
  RED_ON -> (junction 7) : after(switch_time, msec)
  (junction 8) -> (junction 9) [order 2]
  BLUE_ON -> (junction 9) : after(switch_time, msec)
  (junction 7) -> (junction 8) [order 2]
  (junction 7) -> GREEN_ON [order 1] : [green_enable == 1]
  (junction 8) -> BLUE_ON [order 1] : [blue_enable == 1]
  GREEN_ON -> (junction 8) : after(switch_time, msec)
  data: red_out output; red_enable input; blue_enable input; green_enable input; off_time input; switch_time input; blue_out output; green_out output

== stateflow chart Assignment_2_PacemakerProj/AOO/VOO State Diagram ==
  state NO_PACE
    entry:
    s_paceStart = true;
  state PACE
    entry:
    s_paceStart = false;
  (default) -> NO_PACE
  PACE -> NO_PACE : after(p_lowrateInterval, msec)
  NO_PACE -> PACE : after(1, msec)
  data: p_lowrateInterval input; s_paceStart output

== matlab function Assignment_2_PacemakerProj/Decode p_pacingMode ==
  data: p_pacingMode input; s_offState output; s_AOOState output; s_VOOState output; s_AAIState output; S_VVIState output
function [s_offState,s_AOOState, s_VOOState, s_AAIState, S_VVIState] = decodeInputInteger(p_pacingMode)

stateList = zeros(1,5);

stateList(p_pacingMode + 1) = 1;

s_offState = stateList(1);
s_AOOState = stateList(2);
s_VOOState = stateList(3);
s_AAIState = stateList(4);
S_VVIState = stateList(5);

== stateflow chart Assignment_2_PacemakerProj/Button State Changer/Chart ==
  state zeroState_
    entry:
    s_currentState = 0;
  state oneState
    entry:
    s_currentState = 1;
  note: State Number
      | State Name
      |
      | 0
      | OFF
      |
      | 1
      | AOO
      |
      | 2
      | VOO
      |
      | 3
      | AAI
      |
      | 4
      | VVI
  state fourState
    entry:
    s_currentState = 4;
  state twoState
    entry:
    s_currentState = 2;
  state threeState
    entry:
    s_currentState = 3;
  (default) -> zeroState_
  oneState -> twoState : after(1.3, sec)[s_buttonPress == true]
  fourState -> zeroState_ : after(1.3, sec)[s_buttonPress == true]
  zeroState_ -> oneState : after(1.3, sec)[s_buttonPress == true]
  twoState -> threeState : after(1.3, sec)[s_buttonPress == true]
  threeState -> fourState : after(1.3, sec)[s_buttonPress == true]
  data: s_buttonPress input; s_currentState output
